simulink model "SOGI_FLL"  (R2020b)
settings: Solver=ode3  StartTime=0.0  StopTime=0.5  FixedStep=1e-6  RelTol=1e-3
undefined symbols (not defined in the file): DiscIntNeverNeededParam, Ts
libraries: powerlib_meascontrol x1, pid_lib x1
settings Model: Creator=gc45  LastModifiedBy=Administrator

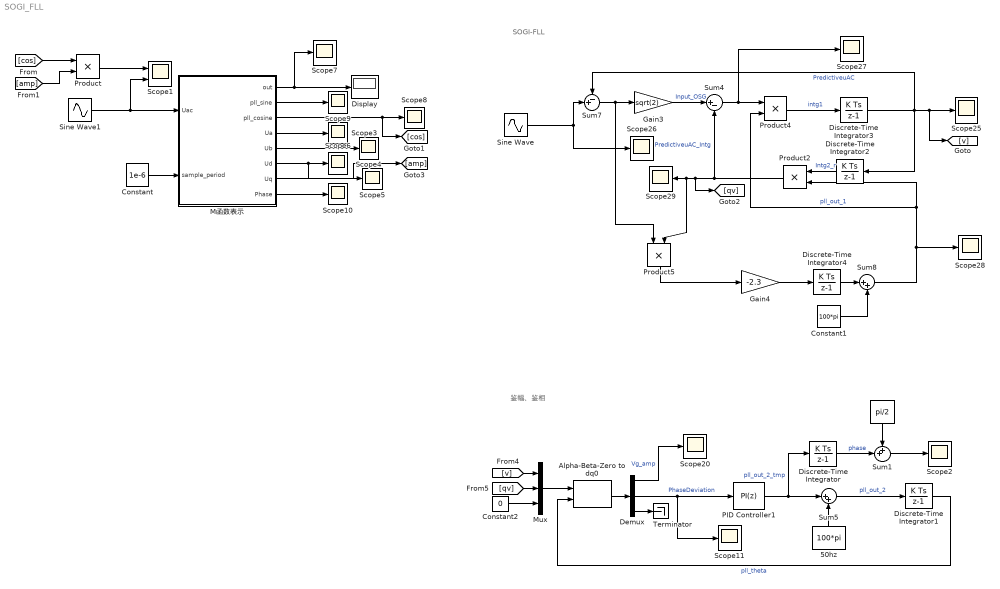
== system SOGI_FLL ==
  note: 鉴幅、鉴相
  note: SOGI-FLL
  " " : Constant  Value=pi/2  SampleTime=Ts
  50hz : Constant  Value=100*pi  SampleTime=Ts
  Alpha-Beta-Zero to dq0 : powerlib_meascontrol/Transformations/Alpha-Beta-Zero to dq0  Alignment=Aligned with phase A axis
  Constant : Constant  Value=1e-6
  Constant1 : Constant  Value=100*pi
  Constant2 : Constant  Value=0
  Demux : Demux  Outputs=3
  Discrete-Time Integrator{,1..4} (5 alike) : DiscreteIntegrator  SampleTime=1e-6  ICPrevOutput=DiscIntNeverNeededParam  ICPrevScaledInput=DiscIntNeverNeededParam
  Display : Display
  Gain3 : Gain  Gain=sqrt(2)
  Gain4 : Gain  Gain=-2.3
  Mux : Mux  Inputs=3
  M函数表示 : MATLAB Function  TreatAsAtomicUnit=on
  PID Controller1 : pid_lib/PID Controller  Controller=PI  Form=Parallel  TimeDomain=Discrete-time  UseExternalTs=off  SampleTime=1e-6  IntegratorMethod=Forward Euler  FilterMethod=Forward Euler  ControllerParametersSource=internal  P=15  I=5  D=0.000000000000000  UseFilter=on  N=99.995000166663857  TunerSelectOption=Transfer Function Based (PID Tuner App)  InitialConditionSource=internal  InitialConditionForIntegrator=0  InitialConditionForFilter=0  DifferentiatorICPrevScaledInput=0  ExternalReset=none  TrackingMode=off  Kt=1  LimitOutput=off  SatLimitsSource=internal  UpperSaturationLimit=inf  LowerSaturationLimit=-inf  LinearizeAsGain=on  AntiWindupMode=none  Kb=1  POutMin=[]  POutMax=[]  IOutMin=[]  IOutMax=[]  DOutMin=[]  DOutMax=[]  NOutMin=[]  NOutMax=[]  SumOutMin=[]  SumOutMax=[]  SaturationOutMin=[]  SaturationOutMax=[]  PParamMin=[]  PParamMax=[]  IParamMin=[]  IParamMax=[]  DParamMin=[]  DParamMax=[]  NParamMin=[]  NParamMax=[]  KbParamMin=[]  KbParamMax=[]  KtParamMin=[]  KtParamMax=[]  KbOutMin=[]  KbOutMax=[]  KtOutMin=[]  KtOutMax=[]  IntegratorOutMin=[]  IntegratorOutMax=[]  FilterOutMin=[]  FilterOutMax=[]  SumI1OutMin=[]  SumI1OutMax=[]  SumI2OutMin=[]  SumI2OutMax=[]  SumI3OutMin=[]  SumI3OutMax=[]  SumI4OutMin=[]  SumI4OutMax=[]  SumDOutMin=[]  SumDOutMax=[]  DifferentiatorOutMin=[]  DifferentiatorOutMax=[]  FilterDiffOutCoefMin=[]  FilterDiffOutCoefMax=[]  ReciprocalOutMin=[]  ReciprocalOutMax=[]  SumDenOutMin=[]  SumDenOutMax=[]  SumNumOutMin=[]  SumNumOutMax=[]  DivideOutMin=[]  DivideOutMax=[]  UdiffTsProdOutMin=[]  UdiffTsProdOutMax=[]  NTsProdOutMin=[]  NTsProdOutMax=[]  UintegralTsProdOutMin=[]  UintegralTsProdOutMax=[]  UngainTsProdOutMin=[]  UngainTsProdOutMax=[]  IntegratorContinuousStateAttributes=''  IntegratorStateMustResolveToSignalObject=off  IntegratorRTWStateStorageClass=Auto  FilterContinuousStateAttributes=''  FilterStateMustResolveToSignalObject=off  FilterRTWStateStorageClass=Auto  ParallelPVariant=InternalParameters  IdealPVariant=Disabled  IVariant=InternalParameters  DVariant=Disabled  IntegratorVariant=Discrete  SatVariant=Disabled  AWVariant=Passthrough  PCopyVariant=Disabled  TRVariant=Disabled  FdbkBlocksVariant=Forward  IdealPFdbkVariant=Disabled  SatFdbkVariant=Disabled  DerivativeFilterVariant=Disabled  NVariant=Disabled  NCopyVariant=Disabled_SignalSpec  FilterICVariant=Disabled  IntegratorICVariant=InternalICs  ExternalResetVariant=Disabled  TRSumVariant=Passthrough  SumFdbkVariant=Disabled  SumVariant=Sum_PI  TsampFilterVariant=InternalTs  TsampNgainVariant=Passthrough  TsampIntegralVariant=Passthrough  ExternalSaturationOutDataTypeStr=Inherit: Same as second input
  Product{,2,4..5} (4 alike) : Product
  Scope1 : Scope  NumInputPorts=2
  Scope{2..11,20,25..29} (16 alike) : Scope
  Sine Wave : Sin  Amplitude=220  Frequency=2*pi*50  Phase=pi/4  SampleTime=1e-6
  Sine Wave1 : Sin  Amplitude=200  Frequency=100*pi  Phase=pi/4  SampleTime=1e-6
  Sum1 : Sum  Inputs=++|
  Sum4 : Sum  Inputs=|+-
  Sum5 : Sum  Inputs=|++
  Sum7 : Sum  Inputs=-+|
  Sum8 : Sum  Inputs=|++
  Terminator : Terminator
  wires:
  Sine Wave1/1 -> M函数表示/1(Uac), Scope1/2
  M函数表示/1(out) -> Scope7/1, Display/1
  Constant/1 -> M函数表示/2(sample_period)
  M函数表示/4(Ua) -> Scope3/1
  M函数表示/5(Ub) -> Scope4/1
  M函数表示/7(Uq) -> Scope5/1
  M函数表示/6(Ud) -> [amp], Scope6/1
  M函数表示/3(pll_cosine) -> [cos], Scope8/1
  M函数表示/2(pll_sine) -> Scope9/1
  M函数表示/8(Phase) -> Scope10/1
  Sine Wave/1 -> Sum7/2, Scope26/1
  Product5/1 -> Gain4/1
  Sum8/1 -> Product4/2, Product2/2, Scope28/1  "pll_out_1"
  Gain3/1 -> Sum4/1  "Input_OSG"
  Sum7/1 -> Product5/1, Gain3/1
  Gain4/1 -> Discrete-Time Integrator4/1
  Discrete-Time Integrator3/1 -> Sum7/1, Discrete-Time Integrator2/1, [v], Scope25/1  "PredictiveuAC"
  Sum4/1 -> Product4/1, Scope27/1
  Discrete-Time Integrator2/1 -> Product2/1  "Intg2_r"
  Constant1/1 -> Sum8/2
  Discrete-Time Integrator4/1 -> Sum8/1
  Product4/1 -> Discrete-Time Integrator3/1  "intg1"
  Product2/1 -> [qv], Product5/2, Scope29/1, Sum4/2  "PredictiveuAC_Intg"
  Alpha-Beta-Zero to dq0/1 -> Demux/1
  Demux/2 -> PID Controller1/1, Scope11/1  "PhaseDeviation"
  Discrete-Time Integrator1/1 -> Alpha-Beta-Zero to dq0/2  "pll_theta"
  Demux/1 -> Scope20/1  "Vg_amp"
  Mux/1 -> Alpha-Beta-Zero to dq0/1
  PID Controller1/1 -> Discrete-Time Integrator/1, Sum5/1  "pll_out_2_tmp"
  [v] -> Mux/1
  [qv] -> Mux/2
  Constant2/1 -> Mux/3
  Sum5/1 -> Discrete-Time Integrator1/1  "pll_out_2"
  Demux/3 -> Terminator/1
  50hz/1 -> Sum5/2
  Discrete-Time Integrator/1 -> Sum1/2  "phase"
  " "/1 -> Sum1/1
  Sum1/1 -> Scope2/1
  [cos] -> Product/1
  [amp] -> Product/2
  Product/1 -> Scope1/1

== matlab function SOGI_FLL/M函数表示 ==
  data: out output; pll_sine output; pll_cosine output; Uac input; sample_period input; Ua output; Ub output; Ud output; Uq output; Phase output
function [out,pll_sine, pll_cosine,Ua,Ub,Ud,Uq,Phase] = SOGI_FLL(Uac, sample_period)

%参数初始化
persistent PredictiveuAC_Intg PredictiveuAC pll_out_1 PhaseDeviation Input_OSG;
persistent pll_Sine pll_Cosine pll_theta Vg_amp PhaseDeviation_Intg pll_out_tmp;
if isempty(pll_out_1)
    PredictiveuAC = 0; %Ualpha
	PredictiveuAC_Intg = 0;%Ubeta
	pll_out_1 = 0;
	PhaseDeviation = 0;
	Input_OSG = 0;
	pll_Sine = 0;
	pll_Cosine = 0;
	pll_theta = 0;
	Vg_amp = 0;
	PhaseDeviation_Intg = 0;
    pll_out_tmp = 0;
end
persistent Intg1 Intg2 Intg2_r Intg3;
if isempty(Intg1)
    Intg1 = 0;
    Intg2 = 0;
    Intg2_r = 0;
    Intg3 = 0;
end
dataType = 'double';
Kp_Predictive = 1.414;%100>>8
Ki_SOGI = 5;
Kp_SOGI = 15;
M = -2.3;
pll_out_2_tmp = 0;
%正交信号发生器环节
   Input_OSG = (Uac-PredictiveuAC) * Kp_Predictive;
   Intg1 = (Input_OSG - PredictiveuAC_Intg) * pll_out_1 * sample_period;
   PredictiveuAC = PredictiveuAC + Intg1;
   Intg2 = PredictiveuAC * sample_period;
   Intg2_r = Intg2_r + Intg2%wky add
   PredictiveuAC_Intg = Intg2_r * pll_out_1;
   Intg3 = (Uac-PredictiveuAC) * PredictiveuAC_Intg * M * sample_period;
   pll_out_tmp = pll_out_tmp + Intg3;
   pll_out_1 = pll_out_tmp + 314.159265358979;
   persistent pll_out_2 phase;
   if isempty(pll_out_2)
    pll_out_2 = 0;
    phase = 0;
   end
%clark变换环节
   PhaseDeviation = -PredictiveuAC * pll_Sine + PredictiveuAC_Intg * pll_Cosine;%q-axis
   Vg_amp = PredictiveuAC * pll_Cosine + (PredictiveuAC_Intg) * pll_Sine;%d-axis
%PI环节
   PhaseDeviation_Intg = PhaseDeviation_Intg + PhaseDeviation * sample_period;
   pll_out_2_tmp = PhaseDeviation_Intg * Ki_SOGI + PhaseDeviation * Kp_SOGI
   phase = phase + pll_out_2_tmp * sample_period;
   pll_out_2 = 314.159265358979 + pll_out_2_tmp;
%限幅环节
 %  if(pll_out > 439)
%        pll_out = 439;
%    end
%    if(pll_out < 251)
%       pll_out = 251;
%    end
    pll_theta = pll_theta + pll_out_2 * sample_period;
    while(pll_theta > 2*pi)
        pll_theta = pll_theta - 2*pi;
    end
    while(pll_theta<0)
        pll_theta = pll_theta + 2*pi;
    end
   out = pll_out_2;
   pll_sine = pll_Sine;
   pll_cosine = pll_Cosine;
   pll_Sine = sin(pll_theta);
   pll_Cosine = cos(pll_theta);
   Ua = PredictiveuAC;
   Ub = PredictiveuAC_Intg;
   Ud = Vg_amp;
   Uq = PhaseDeviation;
   Phase = phase + pi/2;
